simulink model "phase1_LCL_CurRepControl_CIM_adapt"  (R2024a)
settings: Solver=ode23tb  StartTime=0.0  StopTime=3  FixedStep=1e-6  MaxStep=1e-6  RelTol=1e-6
values from neighbouring files (symbols this model uses):
  Cf = 22e-6    (= 2.2e-05)    [phase1_LCL_CurRepControl_CIM_2ndOrder_init.m]
  freq0var = 50    [phase1_LCL_CurRepControl_CIM_2ndOrder_init.m]
  freq2var = 50.5    [phase1_LCL_CurRepControl_CIM_2ndOrder_init.m]
  L1 = 150e-6    (= 0.00015)    [phase1_LCL_CurRepControl_CIM_2ndOrder_init.m]
  L2g = L2+Lg    (= 0.00045)    [phase1_LCL_CurRepControl_CIM_2ndOrder_init.m]
  R1 = 0.045    [phase1_LCL_CurRepControl_CIM_2ndOrder_init.m]
  R2g = R2+Rg    (= 0.135)    [phase1_LCL_CurRepControl_CIM_2ndOrder_init.m]
  Rd = 1    [phase1_LCL_CurRepControl_CIM_2ndOrder_init.m]
  wc = 2*pi*2550    (= 16022.1225333)    [phase1_LCL_CurRepControl_CIM_2ndOrder_init.m]
libraries: spsSeriesRLCBranchLib x6, spsVoltageMeasurementLib x5, spsDiodeLib x4, cstblocks x3, spsDCVoltageSourceLib x2, simulink x2, spsControlledVoltageSourceLib x1, spsCurrentMeasurementLib x1, spsBreakerLib x1, spsPLLLib x1, spsdq0toAlphaBetaZeroLib x1, spsUniversalBridgeLib x1
settings Model: Creator=aleks  LastModifiedBy=aleks
settings DataIOCC: ReturnWorkspaceOutputs=off
settings SimscapeCC: SimscapeLogType=all  SimscapeLogOpenViewer=on  SimscapeLogLimitData=off

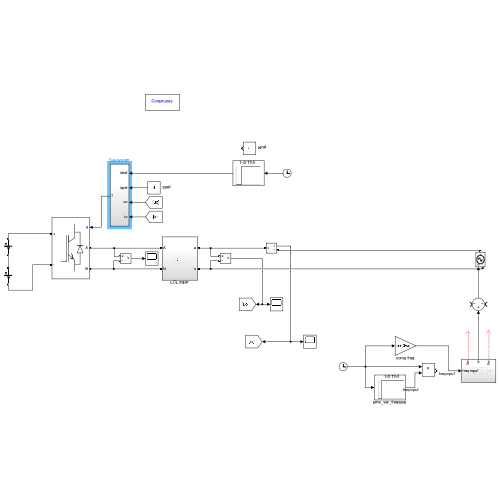
[thumbnail: Simulink's stored preview of the top-level diagram]
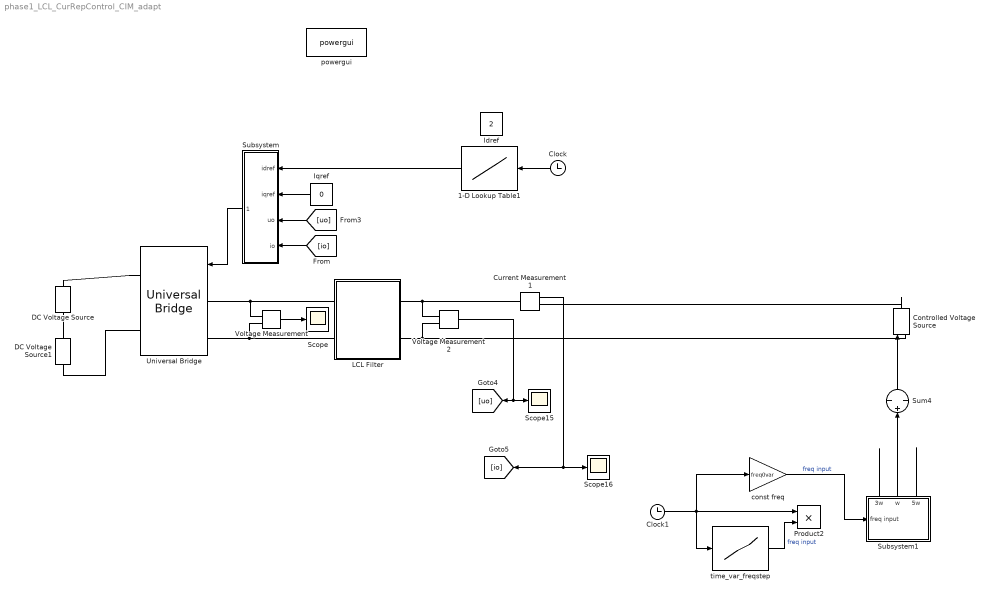
== system phase1_LCL_CurRepControl_CIM_adapt ==
  1-D Lookup Table1 : Lookup_n-D  NumberOfTableDimensions=1  LookupTableObject=''  BreakpointsForDimension1=[0;1.0;1.001;4.5]  BreakpointsForDimension1FirstPoint=10  BreakpointsForDimension2FirstPoint=10  BreakpointsForDimension1Spacing=12  BreakpointsForDimension2Spacing=12  IndexSearchMethod=Linear search  Table=[0;0;2;2]  DiagnosticForOutOfRangeInput=Error  InternalRulePriority=Speed  RndMeth=Simplest
  Clock : Clock
  Clock1 : Clock
  Controlled Voltage Source : spsControlledVoltageSourceLib/Controlled Voltage Source  Initialize=on  Source_Type=AC  Amplitude=0  Phase=0  Frequency=0  Measurements=None
  Current Measurement1 : spsCurrentMeasurementLib/Current Measurement  PhasorSimulation=off  OutputType=Complex  PSBequivalent=0
  DC Voltage Source : spsDCVoltageSourceLib/DC Voltage Source  Amplitude=20  Measurements=None
  DC Voltage Source1 : spsDCVoltageSourceLib/DC Voltage Source  Amplitude=20  Measurements=None
  Idref : Constant  Value=2
  Iqref : Constant  Value=0
  LCL Filter : Subsystem
  Product2 : Product
  Scope : Scope
  Scope15 : Scope
  Scope16 : Scope
  Subsystem : Subsystem
  Subsystem1 : Subsystem
      settings: PortSchema="{\"entries\":[{\"content\":{\"sides\":[{\"content\":{\"connectorIds\":[\"In1\"]},\"type\":\"ConnectorPlacement.EquallySpacedRectSide\",\"uuid\":\"8bb38228-3bfd-4ae6-808e-88de23dff197\"},{\"content\":{\"side\":\"RIGHT\"},\"type\":\"ConnectorPlacement.EquallySpacedRectSide\",\"uuid\":\"838e29f9-37df-4c86-a8f7-90e289e1c513\"},{\"content\":{\"connectorIds\":[\"Out1\",\"Out2\",\"Out3\"],\"side\":\"TOP\"},\"type\":\"ConnectorPlacement.EquallySpacedRectSide\",\"uuid\":\"6e4fecd3-8130-46cd-a081-09e68c069565\"}]},\"type\":\"ConnectorPlacement.EquallySpacedConnector\",\"uuid\":\"764d7bec-48d4-42ac-bbe4-5dd81e7c6ed5\"}],\"packageUris\":[\"http://schema.mathworks.com/mf0/Connector/R2020b\"],\"version\":\"1.0\"}"
  Sum4 : Sum  Inputs=-|+|-
  Universal Bridge : spsUniversalBridgeLib/Universal Bridge  Arms=2  SnubberResistance=1e5  SnubberCapacitance=inf  Device=IGBT / Diodes  Ron=1e-3  Lon=0  ForwardVoltages="[  0  0  ]"  ForwardVoltage=0  GTOparameters=[ 10e-6 , 20e-6 ]  IGBTparameters=[ 1e-6 , 2e-6 ]  Measurements=None  Measurements_2=None  converterType=Rectifier
  Voltage Measurement : spsVoltageMeasurementLib/Voltage Measurement  PhasorSimulation=off  OutputType=Complex  PSBequivalent=0
  Voltage Measurement2 : spsVoltageMeasurementLib/Voltage Measurement  PhasorSimulation=off  OutputType=Complex  PSBequivalent=0
  const freq : Gain  Gain=freq0var
  powergui : spspowerguiLib/powergui  Priority=1  SimulationMode=Continuous  SampleTime=10e-6  frequency=60  Iterations=50  frequencyindice=0  Pbase=100e6  ErrMax=1e-4  UnitsV=kV  UnitsW=MW  buscounter=0  FunctionMessages=off  echomessages=off  EnableUseOfTLC=off  CurrentSourceSwitches=off  DisableSnubberDevices=off  DisableRonSwitches=off  DisableVfSwitches=off  DisplayEquations=off  AutomaticDiscreteSolvers=off  SolverType=Tustin/Backward Euler (TBE)  Interpol=off  ExternalGateDelay=off  methode=off  Ts=100  x0status=blocks  SPID=on  SwTol=0  HookPort=off  NonlinearTolerance=1e-4  nMaxIteration=100  ContinueOnMaxIteration=off  RestoreLinks=warning  ResistiveCurrentMeasurement=off  Frange=[0:2:500]  Ylog=off  Xlog=on  ShowGrid=off  save=off  variable=ZData  structure=0  ZoomFFT=off  StartTime=0.0  cycles=1  DisplayStyle=1  fundamental=60  FreqAxis=off  MaxFrequency=1000  frequencyindicesteady=1  RmsSteady=1  display=off
  time_var_freqstep : Lookup_n-D  NumberOfTableDimensions=1  LookupTableObject=''  BreakpointsForDimension1=[0;0.2;0.201;1.5]  BreakpointsForDimension1FirstPoint=10  BreakpointsForDimension2FirstPoint=10  BreakpointsForDimension1Spacing=12  BreakpointsForDimension2Spacing=12  IndexSearchMethod=Linear search  Table=[freq0var;freq0var;freq2var;freq2var]  DiagnosticForOutOfRangeInput=Error  InternalRulePriority=Speed  RndMeth=Simplest
  wires:
  Voltage Measurement/1 -> Scope/1
  Subsystem/1(1) -> Universal Bridge/1
  [io] -> Subsystem/4(io)
  [uo] -> Subsystem/3(uo)
  Voltage Measurement2/1 -> [uo], Scope15/1
  Current Measurement1/1 -> Scope16/1, [io]
  Sum4/1 -> Controlled Voltage Source/1
  1-D Lookup Table1/1 -> Subsystem/1(idref)
  Clock/1 -> 1-D Lookup Table1/1
  Iqref/1 -> Subsystem/2(iqref)
  Clock1/1 -> time_var_freqstep/1, Product2/1, const freq/1
  const freq/1 -> Subsystem1/1(freq input)  "freq input"
  Subsystem1/1(3w) -> ?
  Subsystem1/2(w) -> Sum4/2
  Subsystem1/3(5w) -> ?
  time_var_freqstep/1 -> Product2/2  "freq input"
  connections:
  Universal Bridge/RConn1 -- DC Voltage Source/RConn1
  Universal Bridge/RConn2 -- DC Voltage Source1/LConn1
  Voltage Measurement/LConn1 -- LCL Filter/LConn1 -- Universal Bridge/LConn1
  Voltage Measurement2/LConn2 -- Controlled Voltage Source/LConn1 -- LCL Filter/RConn2
  DC Voltage Source/LConn1 -- DC Voltage Source1/RConn1
  Voltage Measurement2/LConn1 -- LCL Filter/RConn1 -- Current Measurement1/LConn1
  Controlled Voltage Source/RConn1 -- Current Measurement1/RConn1
  Voltage Measurement/LConn2 -- LCL Filter/LConn2 -- Universal Bridge/LConn2

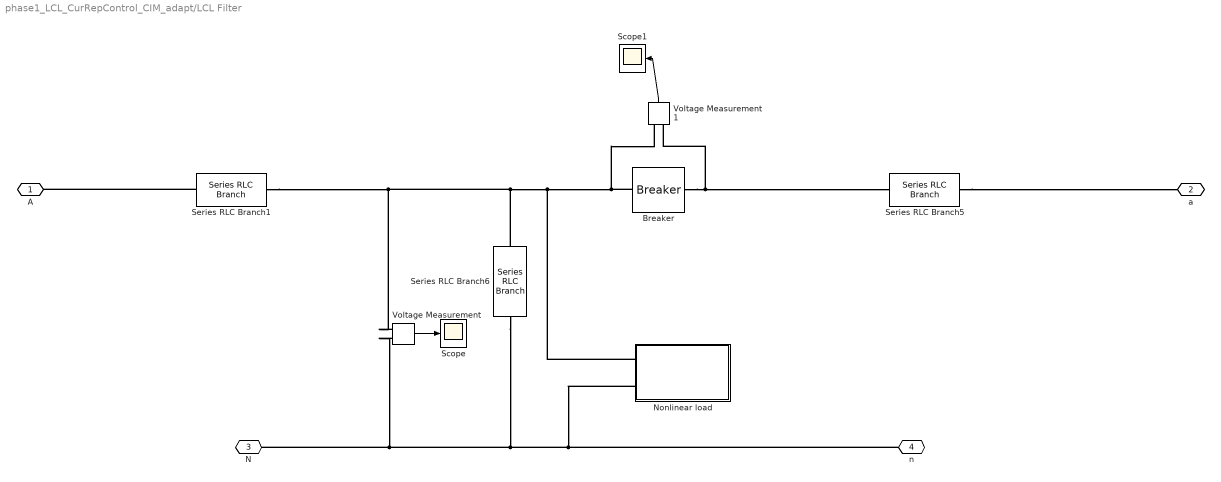
== system phase1_LCL_CurRepControl_CIM_adapt/LCL Filter ==
  Breaker : spsBreakerLib/Breaker  InitialState=0  SwitchingTimes=[0]  External=off  BreakerResistance=0.0001  SnubberResistance=1e8  SnubberCapacitance=inf  Measurements=None  MoreParameters=on  NoBreakLoop=off
  Nonlinear load : Subsystem
  Scope : Scope
  Scope1 : Scope
  Series RLC Branch1 : spsSeriesRLCBranchLib/Series RLC Branch  LConnTagsString=__new0  RConnTagsString=__new0  BranchType=RL  Resistance=R1  Inductance=L1  SetiL0=off  InitialCurrent=0  Capacitance=1e-6  Setx0=off  InitialVoltage=0  Measurements=None
  Series RLC Branch5 : spsSeriesRLCBranchLib/Series RLC Branch  LConnTagsString=__new0  RConnTagsString=__new0  BranchType=RL  Resistance=R2g  Inductance=L2g  SetiL0=off  InitialCurrent=0  Capacitance=1e-6  Setx0=off  InitialVoltage=0  Measurements=None
  Series RLC Branch6 : spsSeriesRLCBranchLib/Series RLC Branch  LConnTagsString=__new0  RConnTagsString=__new0  BranchType=RC  Resistance=Rd  Inductance=500e-6  SetiL0=off  InitialCurrent=0  Capacitance=Cf  Setx0=off  InitialVoltage=0  Measurements=None
  Voltage Measurement : spsVoltageMeasurementLib/Voltage Measurement  PhasorSimulation=off  OutputType=Complex  PSBequivalent=0
  Voltage Measurement1 : spsVoltageMeasurementLib/Voltage Measurement  PhasorSimulation=off  OutputType=Complex  PSBequivalent=0
  A : PMIOPort  Side=Left
  a : PMIOPort  Port=2  Side=Right
  N : PMIOPort  Port=3  Side=Left
  n : PMIOPort  Port=4  Side=Right
  wires:
  Voltage Measurement1/1 -> Scope1/1
  Voltage Measurement/1 -> Scope/1
  connections:
  Voltage Measurement/LConn2 -- N/RConn1 -- Nonlinear load/LConn2 -- n/RConn1 -- Series RLC Branch6/LConn1
  Series RLC Branch1/RConn1 -- Series RLC Branch6/RConn1 -- Nonlinear load/LConn1 -- Voltage Measurement1/LConn2 -- Breaker/LConn1 -- Voltage Measurement/LConn1
  Voltage Measurement1/LConn1 -- Breaker/RConn1 -- Series RLC Branch5/LConn1
  Series RLC Branch1/LConn1 -- A/RConn1
  Series RLC Branch5/RConn1 -- a/RConn1

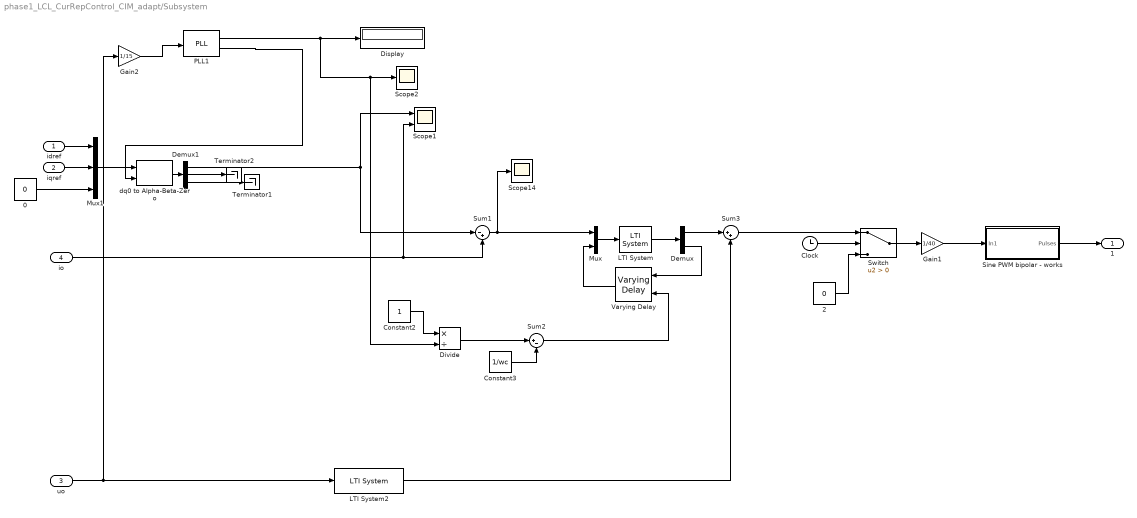
== system phase1_LCL_CurRepControl_CIM_adapt/Subsystem ==
  idref : Inport
  iqref : Inport  Port=2
  uo : Inport  Port=3
  io : Inport  Port=4
  0 : Constant  Value=0
  2 : Constant  Value=0
  Clock : Clock
  Constant2 : Constant
  Constant3 : Constant  Value=1/wc
  Demux : Demux  Outputs=2
  Demux1 : Demux  Outputs=3
  Display : Display
  Divide : Product  Inputs=*/
  Gain1 : Gain  Gain=1/40
  Gain2 : Gain  Gain=1/15
  LTI System : cstblocks/LTI System  sys=Psi_tf  IC=[]  PadeOrder=0
  LTI System2 : cstblocks/LTI System  sys=Gfffilter  IC=[]  PadeOrder=0
  Mux : Mux  Inputs=2
  Mux1 : Mux  Inputs=3
  PLL1 : spsPLLLib/PLL  Fmin=49  Par_Init=[0, freq2var]  ParK=[180, 3200, 1]  TcD=1e-4  MaxRateChangeFreq=2  FilterCutOffFreq=25  Ts=0  AGC=on
      settings: LibrarySourceBlock=sps_lib/Control/PLL
  Scope1 : Scope  NumInputPorts=2
  Scope14 : Scope
  Scope2 : Scope
  Sine PWM bipolar - works : Subsystem
  Sum1 : Sum  Inputs=|-+
  Sum2 : Sum  Inputs=|+-
  Sum3 : Sum  Inputs=|++
  Switch : Switch  Criteria=u2 > Threshold  SaturateOnIntegerOverflow=off  InputSameDT=off
  Terminator1 : Terminator
  Terminator2 : Terminator
  Varying Delay : cstblocks/Linear Parameter Varying/Varying Delay  Td=tau_d  TdMax=10  TdMin=0  TdFixed=[]  u0=0  bufsize=1024  FixedBuffer=off  PadeOrder=0
  dq0 to Alpha-Beta-Zero : spsdq0toAlphaBetaZeroLib/dq0 to Alpha-Beta-Zero  Alignment=90 degrees behind phase A axis
  1 : Outport
  wires:
  Demux1/1 -> Scope1/1, Sum1/1
  io/1 -> Scope1/2, Sum1/2
  Sine PWM bipolar - works/1(Pulses) -> 1/1
  Gain1/1 -> Sine PWM bipolar - works/1(In1)
  Sum3/1 -> Switch/1
  Sum1/1 -> Mux/1, Scope14/1
  Demux/1 -> Sum3/1
  Varying Delay/1 -> Mux/2
  Mux/1 -> LTI System/1
  Demux/2 -> Varying Delay/1
  LTI System/1 -> Demux/1
  LTI System2/1 -> Sum3/2
  Constant2/1 -> Divide/1
  Constant3/1 -> Sum2/2
  Sum2/1 -> Varying Delay/2
  PLL1/2 -> dq0 to Alpha-Beta-Zero/2
  dq0 to Alpha-Beta-Zero/1 -> Demux1/1
  Mux1/1 -> dq0 to Alpha-Beta-Zero/1
  idref/1 -> Mux1/1
  0/1 -> Mux1/3
  Demux1/2 -> Terminator2/1
  iqref/1 -> Mux1/2
  Demux1/3 -> Terminator1/1
  Clock/1 -> Switch/2
  2/1 -> Switch/3
  Divide/1 -> Sum2/1
  Switch/1 -> Gain1/1
  uo/1 -> Gain2/1, LTI System2/1
  Gain2/1 -> PLL1/1
  PLL1/1 -> Divide/2, Scope2/1, Display/1

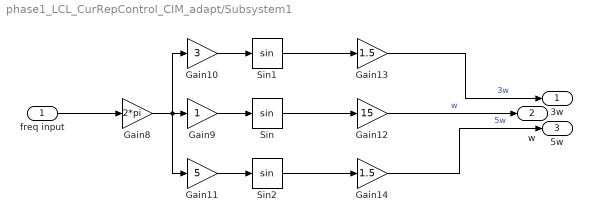
== system phase1_LCL_CurRepControl_CIM_adapt/Subsystem1 ==
  freq input : Inport
  Gain10 : Gain  Gain=3
  Gain11 : Gain  Gain=5
  Gain12 : Gain  Gain=15
  Gain13 : Gain  Gain=1.5
  Gain14 : Gain  Gain=1.5
  Gain8 : Gain  Gain=2*pi
  Gain9 : Gain
  Sin : Trigonometry
  Sin1 : Trigonometry
  Sin2 : Trigonometry
  3w : Outport
  w : Outport  Port=2
  5w : Outport  Port=3
  wires:
  Gain14/1 -> 5w/1  "5w"
  Gain12/1 -> w/1  "w"
  Gain9/1 -> Sin/1
  freq input/1 -> Gain8/1
  Sin/1 -> Gain12/1
  Gain13/1 -> 3w/1  "3w"
  Sin1/1 -> Gain13/1
  Gain8/1 -> Gain11/1, Gain10/1, Gain9/1
  Gain10/1 -> Sin1/1
  Gain11/1 -> Sin2/1
  Sin2/1 -> Gain14/1

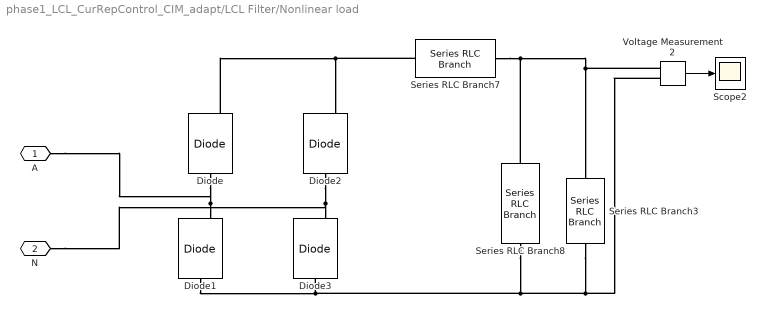
== system phase1_LCL_CurRepControl_CIM_adapt/LCL Filter/Nonlinear load ==
  Diode{,1..3} (4 alike) : spsDiodeLib/Diode  Ron=0.001  Lon=0  Vf=0.8  IC=0  UseSnubber=0  Rs=500  Cs=250e-9  Measurements=on
  Scope2 : Scope
  Series RLC Branch3 : spsSeriesRLCBranchLib/Series RLC Branch  LConnTagsString=__new0  RConnTagsString=__new0  BranchType=R  Resistance=20  Inductance=500e-6  SetiL0=off  InitialCurrent=0  Capacitance=1e-6  Setx0=off  InitialVoltage=0  Measurements=None
  Series RLC Branch7 : spsSeriesRLCBranchLib/Series RLC Branch  LConnTagsString=__new0  RConnTagsString=__new0  BranchType=RL  Resistance=R1  Inductance=L1  SetiL0=off  InitialCurrent=0  Capacitance=1e-6  Setx0=off  InitialVoltage=0  Measurements=None
  Series RLC Branch8 : spsSeriesRLCBranchLib/Series RLC Branch  LConnTagsString=__new0  RConnTagsString=__new0  BranchType=RC  Resistance=0  Inductance=500e-6  SetiL0=off  InitialCurrent=0  Capacitance=1e-3  Setx0=off  InitialVoltage=0  Measurements=None
  Voltage Measurement2 : spsVoltageMeasurementLib/Voltage Measurement  PhasorSimulation=off  OutputType=Complex  PSBequivalent=0
  A : PMIOPort  Side=Left
  N : PMIOPort  Port=2  Side=Left
  wires:
  Voltage Measurement2/1 -> Scope2/1
  connections:
  Series RLC Branch8/RConn1 -- Series RLC Branch7/RConn1 -- Voltage Measurement2/LConn1 -- Series RLC Branch3/RConn1
  Diode/RConn1 -- Diode2/RConn1 -- Series RLC Branch7/LConn1
  Diode2/LConn1 -- Diode3/RConn1 -- N/RConn1
  Series RLC Branch3/LConn1 -- Series RLC Branch8/LConn1 -- Diode1/LConn1 -- Diode3/LConn1 -- Voltage Measurement2/LConn2
  Diode1/RConn1 -- Diode/LConn1 -- A/RConn1

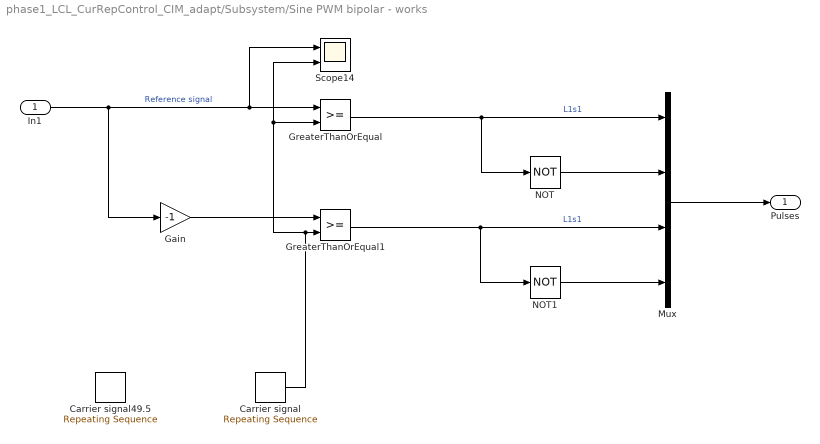
== system phase1_LCL_CurRepControl_CIM_adapt/Subsystem/Sine PWM bipolar - works ==
  In1 : Inport
  Carrier signal : simulink/Sources/Repeating Sequence  rep_seq_t=[0 1/24000 1/12000]  rep_seq_y=[-1 1 -1]
  Carrier signal49.5 : simulink/Sources/Repeating Sequence  rep_seq_t=[0 1/23760 1/11880]  rep_seq_y=[-1 1 -1]
  Gain : Gain  Gain=-1
  GreaterThanOrEqual : RelationalOperator  OutDataTypeStr=boolean  RndMeth=Simplest  InputSameDT=off
  GreaterThanOrEqual1 : RelationalOperator  OutDataTypeStr=boolean  RndMeth=Simplest  InputSameDT=off
  Mux : Mux
  NOT : Logic  Operator=NOT  IconShape=distinctive  AllPortsSameDT=off  OutDataTypeStr=boolean
  NOT1 : Logic  Operator=NOT  IconShape=distinctive  AllPortsSameDT=off  OutDataTypeStr=boolean
  Scope14 : Scope  NumInputPorts=2
  Pulses : Outport
  wires:
  Mux/1 -> Pulses/1
  In1/1 -> Scope14/1, GreaterThanOrEqual/1, Gain/1  "Reference signal"
  Carrier signal/1 -> Scope14/2, GreaterThanOrEqual/2, GreaterThanOrEqual1/2
  GreaterThanOrEqual/1 -> NOT/1, Mux/1  "L1s1"
  Gain/1 -> GreaterThanOrEqual1/1
  NOT/1 -> Mux/2
  GreaterThanOrEqual1/1 -> NOT1/1, Mux/3  "L1s1"
  NOT1/1 -> Mux/4
